simulink model "ex3"  (R2021b)
settings: Solver=VariableStepAuto  StartTime=0.0  StopTime=10.0  RelTol=1e-3

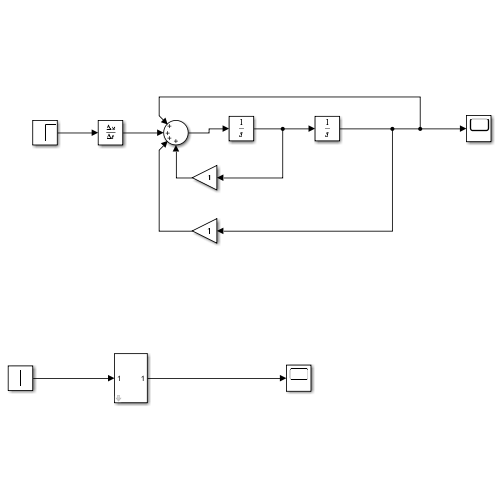
[thumbnail: Simulink's stored preview of the top-level diagram]
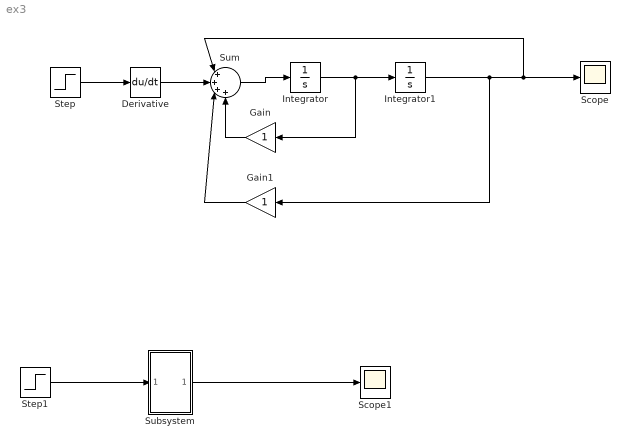
== system ex3 ==
  Derivative : Derivative
  Gain : Gain
  Gain1 : Gain
  Integrator : Integrator
  Integrator1 : Integrator
  Scope : Scope
  Scope1 : Scope
  Step : Step  SampleTime=0
  Step1 : Step  SampleTime=0
  Subsystem : Subsystem  mask{a=3}
      mask Callback a:
      | if str2num(get_param(gcb,'a'))>4
      |     error('Eroare');
      | end
      | 
      | if str2num(get_param(gcb,'a'))<2
      |     error('Eroare');
      | end
  Sum : Sum  Inputs=|++++
  wires:
  Derivative/1 -> Sum/2
  Gain1/1 -> Sum/3
  Gain/1 -> Sum/4
  Integrator1/1 -> Gain1/1, Sum/1, Scope/1
  Step/1 -> Derivative/1
  Integrator/1 -> Gain/1, Integrator1/1
  Sum/1 -> Integrator/1
  Step1/1 -> Subsystem/1(In1)
  Subsystem/1(Out1) -> Scope1/1

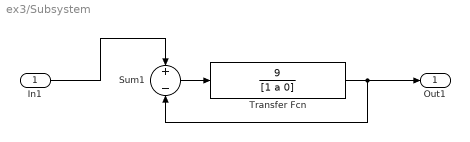
== system ex3/Subsystem ==
  In1 : Inport
  Sum1 : Sum  Inputs=+-
  Transfer Fcn : TransferFcn  Numerator=[9]  Denominator=[1 a 0]
  Out1 : Outport
  wires:
  Sum1/1 -> Transfer Fcn/1
  In1/1 -> Sum1/1
  Transfer Fcn/1 -> Out1/1, Sum1/2
